simulink model "example8_1"  (R2022b)
settings: Solver=VariableStepAuto  StartTime=0.0  StopTime=10.0  RelTol=1e-3
undefined symbols (not defined in the file): a
settings Model: Creator=eechris  LastModifiedBy=eechris

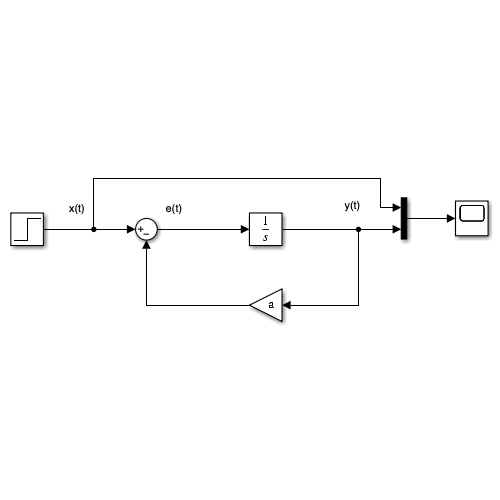
[thumbnail: Simulink's stored preview of the top-level diagram]
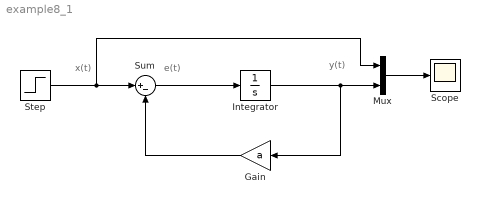
== system example8_1 ==
  note: x(t)
  note: y(t)
  note: e(t)
  Gain : Gain  Gain=a
  Integrator : Integrator
  Mux : Mux  Inputs=2
  Scope : Scope
  Step : Step  SampleTime=0
  Sum : Sum  Inputs=|+-
  wires:
  Integrator/1 -> Mux/2, Gain/1
  Sum/1 -> Integrator/1
  Gain/1 -> Sum/2
  Step/1 -> Mux/1, Sum/1
  Mux/1 -> Scope/1
